simulink subsystem "h_bridge"  (R2023a)
settings: Solver=VariableStepAuto  StartTime=0.0  StopTime=10.0  RelTol=1e-3
libraries: fl_lib x6, nesl_utility x3
settings Model: Creator=motya  LastModifiedBy=motya

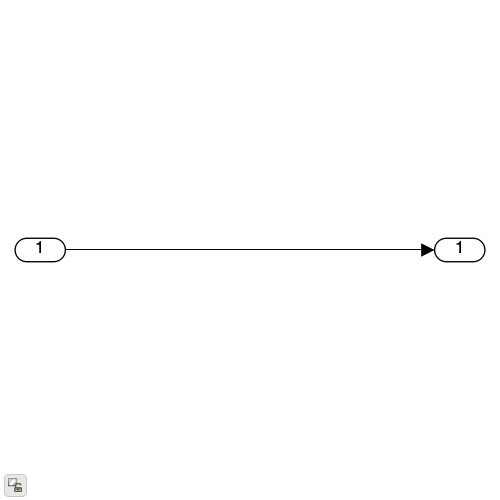
[thumbnail: Simulink's stored preview of the top-level diagram]
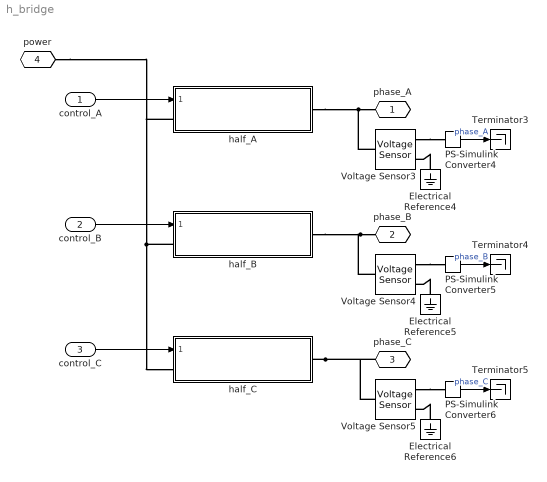
== system h_bridge ==
  control_A : Inport
  control_B : Inport  Port=2
  control_C : Inport  Port=3
  Electrical Reference4 : fl_lib/Electrical/Electrical Elements/Electrical Reference
  Electrical Reference5 : fl_lib/Electrical/Electrical Elements/Electrical Reference
  Electrical Reference6 : fl_lib/Electrical/Electrical Elements/Electrical Reference
  PS-Simulink Converter4 : nesl_utility/PS-Simulink Converter  PhysicalDomain=network_engine_domain  SubClassName=ps_output  LeftPortType=input  RightPortType=output  PseudoPeriodic=off  Frequencies=[]  VectorFormat=inherit  Unit=V  AffineConversion=on
  PS-Simulink Converter5 : nesl_utility/PS-Simulink Converter  PhysicalDomain=network_engine_domain  SubClassName=ps_output  LeftPortType=input  RightPortType=output  PseudoPeriodic=off  Frequencies=[]  VectorFormat=inherit  Unit=V  AffineConversion=on
  PS-Simulink Converter6 : nesl_utility/PS-Simulink Converter  PhysicalDomain=network_engine_domain  SubClassName=ps_output  LeftPortType=input  RightPortType=output  PseudoPeriodic=off  Frequencies=[]  VectorFormat=inherit  Unit=V  AffineConversion=on
  Terminator3 : Terminator
  Terminator4 : Terminator
  Terminator5 : Terminator
  Voltage Sensor3 : fl_lib/Electrical/Electrical Sensors/Voltage Sensor
  Voltage Sensor4 : fl_lib/Electrical/Electrical Sensors/Voltage Sensor
  Voltage Sensor5 : fl_lib/Electrical/Electrical Sensors/Voltage Sensor
  half_A : Subsystem  ReferencedSubsystem=half_bridge
  half_B : Subsystem  ReferencedSubsystem=half_bridge
  half_C : Subsystem  ReferencedSubsystem=half_bridge
  phase_A : PMIOPort  Side=Right
  phase_B : PMIOPort  Port=2  Side=Right
  phase_C : PMIOPort  Port=3  Side=Right
  power : PMIOPort  Port=4  Side=Left
  wires:
  PS-Simulink Converter4/1 -> Terminator3/1  "phase_A"
  PS-Simulink Converter5/1 -> Terminator4/1  "phase_B"
  PS-Simulink Converter6/1 -> Terminator5/1  "phase_C"
  control_A/1 -> half_A/1
  control_B/1 -> half_B/1
  control_C/1 -> half_C/1
  connections:
  half_A/RConn1 -- phase_A/RConn1 -- Voltage Sensor3/LConn1
  phase_B/RConn1 -- Voltage Sensor4/LConn1 -- half_B/RConn1
  half_C/RConn1 -- Voltage Sensor5/LConn1 -- phase_C/RConn1
  half_B/LConn1 -- half_C/LConn1 -- half_A/LConn1 -- power/RConn1
  Electrical Reference4/LConn1 -- Voltage Sensor3/RConn2
  Voltage Sensor3/RConn1 -- PS-Simulink Converter4/LConn1
  Electrical Reference5/LConn1 -- Voltage Sensor4/RConn2
  Voltage Sensor4/RConn1 -- PS-Simulink Converter5/LConn1
  Electrical Reference6/LConn1 -- Voltage Sensor5/RConn2
  Voltage Sensor5/RConn1 -- PS-Simulink Converter6/LConn1
